simulink model "primer2"  (R2014a)
settings: Solver=ode45  StartTime=0.0  StopTime=50.0  RelTol=1e-3
undefined symbols (not defined in the file): des, gcbh
settings Model: Creator=Student  LastModifiedBy=almi0
settings OptimizationCC: ExpressionDepthLimit=2147483647
settings DebuggingCC: UnderspecifiedInitializationDetection=Classic  StateNameClashWarn=warning

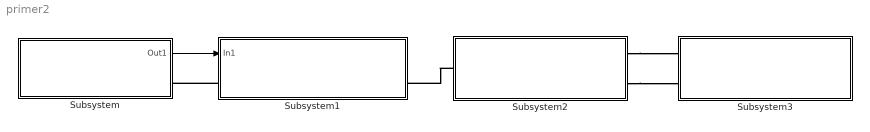
== system primer2 ==
  Subsystem : Subsystem
  Subsystem1 : Subsystem
  Subsystem2 : Subsystem
  Subsystem3 : Subsystem
  wires:
  Subsystem/1(Out1) -> Subsystem1/1(In1)
  connections:
  Subsystem1/LConn1 -- Subsystem/RConn1
  Subsystem2/LConn1 -- Subsystem1/RConn2
  Subsystem2/RConn1 -- Subsystem3/LConn1
  Subsystem2/RConn2 -- Subsystem3/LConn2

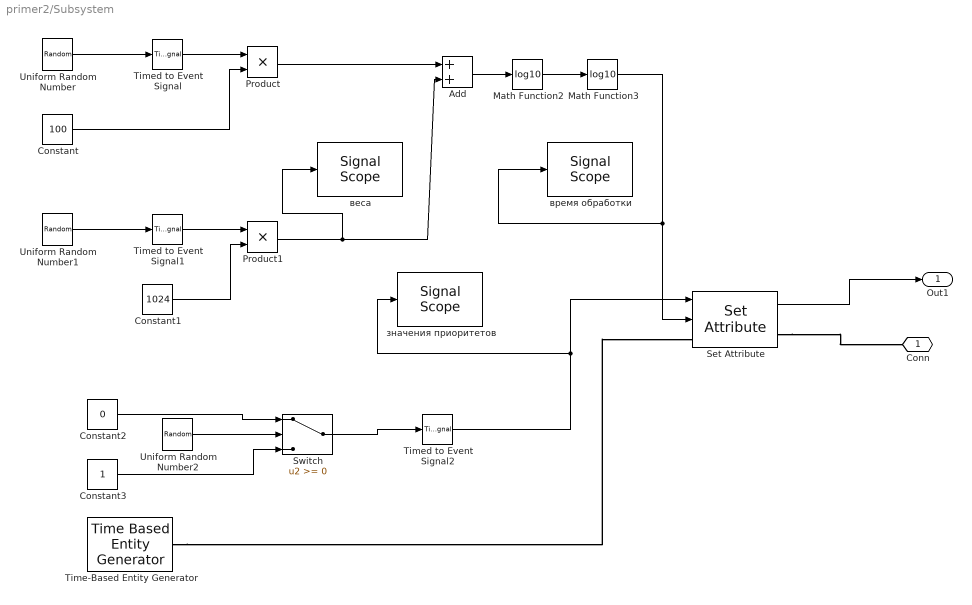
== system primer2/Subsystem ==
  Add : Sum
  Constant : Constant  Value=100
  Constant1 : Constant  Value=1024
  Constant2 : Constant  Value=0
  Constant3 : Constant
  Math Function2 : Math  Operator=log10  SaturateOnIntegerOverflow=on
  Math Function3 : Math  Operator=log10  SaturateOnIntegerOverflow=on
  Product : Product  RndMeth=Zero
  Product1 : Product  RndMeth=Zero
  Set Attribute : SetAttribute  AttributeName=Priority|ServTime  AttributeFrom=Signal port|Signal port  AttributeValue=1|1  AttributeTreatAsVector=1|1  StatNumberDeparted=on  EvaluatedAttributeValue={ [];[]}
      settings: InputPortMap=u0,u1
  Switch : Switch
  Time-Based Entity Generator : TimeBasedEntityGenerator
  Timed to Event Signal : TimedToEventSignal
  Timed to Event Signal1 : TimedToEventSignal
  Timed to Event Signal2 : TimedToEventSignal
  Uniform Random Number : UniformRandomNumber  Minimum=0  SampleTime=0.1
  Uniform Random Number1 : UniformRandomNumber  Minimum=0  SampleTime=0.1
  Uniform Random Number2 : UniformRandomNumber  Minimum=0  SampleTime=0.1
  веса : SignalScope  LoadFcn=des.scope.CallbackSupport('seLoadFcn',gcbh)  StartFcn=des.scope.CallbackSupport('seStartFcn',gcbh)  StopFcn=des.scope.CallbackSupport('seStopFcn',gcbh)
      settings: CopyFcn=des.scope.CallbackSupport('seCopyFcn',gcbh)  DeleteFcn=des.scope.CallbackSupport('seDeleteFcn',gcbh)  PreSaveFcn=des.scope.CallbackSupport('sePreSaveFcn',gcbh)  NameChangeFcn=des.scope.CallbackSupport('seNameChangeFcn',gcbh)  OpenFcn=des.scope.CallbackSupport('seOpenFcn',gcbh)
  время обработки : SignalScope  LoadFcn=des.scope.CallbackSupport('seLoadFcn',gcbh)  StartFcn=des.scope.CallbackSupport('seStartFcn',gcbh)  StopFcn=des.scope.CallbackSupport('seStopFcn',gcbh)  ShowCountPlotted=on
      settings: CopyFcn=des.scope.CallbackSupport('seCopyFcn',gcbh)  DeleteFcn=des.scope.CallbackSupport('seDeleteFcn',gcbh)  PreSaveFcn=des.scope.CallbackSupport('sePreSaveFcn',gcbh)  NameChangeFcn=des.scope.CallbackSupport('seNameChangeFcn',gcbh)  OpenFcn=des.scope.CallbackSupport('seOpenFcn',gcbh)
  значения приоритетов : SignalScope  LoadFcn=des.scope.CallbackSupport('seLoadFcn',gcbh)  StartFcn=des.scope.CallbackSupport('seStartFcn',gcbh)  StopFcn=des.scope.CallbackSupport('seStopFcn',gcbh)
      settings: CopyFcn=des.scope.CallbackSupport('seCopyFcn',gcbh)  DeleteFcn=des.scope.CallbackSupport('seDeleteFcn',gcbh)  PreSaveFcn=des.scope.CallbackSupport('sePreSaveFcn',gcbh)  NameChangeFcn=des.scope.CallbackSupport('seNameChangeFcn',gcbh)  OpenFcn=des.scope.CallbackSupport('seOpenFcn',gcbh)
  Conn : PMIOPort  Port=1  Side=Right
  Out1 : Outport
  wires:
  Switch/1 -> Timed to Event Signal2/1
  Constant2/1 -> Switch/1
  Set Attribute/1 -> Out1/1
  Constant/1 -> Product/2
  Uniform Random Number/1 -> Timed to Event Signal/1
  Math Function2/1 -> Math Function3/1
  Timed to Event Signal/1 -> Product/1
  Product1/1 -> веса/1, Add/2
  Product/1 -> Add/1
  Timed to Event Signal1/1 -> Product1/1
  Constant1/1 -> Product1/2
  Uniform Random Number1/1 -> Timed to Event Signal1/1
  Add/1 -> Math Function2/1
  Constant3/1 -> Switch/3
  Uniform Random Number2/1 -> Switch/2
  Timed to Event Signal2/1 -> Set Attribute/1, значения приоритетов/1
  Math Function3/1 -> время обработки/1, Set Attribute/2
  connections:
  Time-Based Entity Generator/RConn1 -- Set Attribute/LConn1
  Set Attribute/RConn1 -- Conn/RConn1

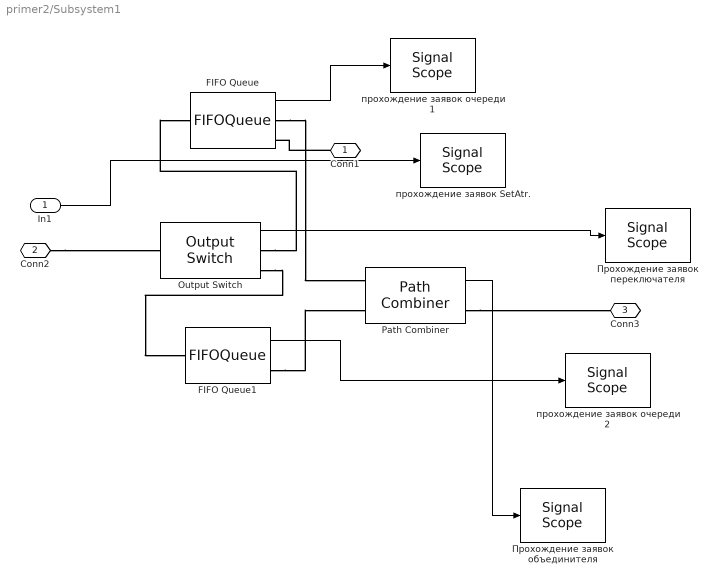
== system primer2/Subsystem1 ==
  In1 : Inport
  FIFO Queue : FIFOQueue  EnableTOPort=on  StatNumberDeparted=on
  FIFO Queue1 : FIFOQueue  StatNumberDeparted=on
  Output Switch : OutputSwitch  NumberOutputPorts=2  StatNumberDeparted=on
  Path Combiner : PathCombiner  NumberInputPorts=2  StatNumberDeparted=on
  Прохождение заявок объединителя : SignalScope  LoadFcn=des.scope.CallbackSupport('seLoadFcn',gcbh)  StartFcn=des.scope.CallbackSupport('seStartFcn',gcbh)  StopFcn=des.scope.CallbackSupport('seStopFcn',gcbh)
      settings: CopyFcn=des.scope.CallbackSupport('seCopyFcn',gcbh)  DeleteFcn=des.scope.CallbackSupport('seDeleteFcn',gcbh)  PreSaveFcn=des.scope.CallbackSupport('sePreSaveFcn',gcbh)  NameChangeFcn=des.scope.CallbackSupport('seNameChangeFcn',gcbh)  OpenFcn=des.scope.CallbackSupport('seOpenFcn',gcbh)
  Прохождение заявок переключателя : SignalScope  LoadFcn=des.scope.CallbackSupport('seLoadFcn',gcbh)  StartFcn=des.scope.CallbackSupport('seStartFcn',gcbh)  StopFcn=des.scope.CallbackSupport('seStopFcn',gcbh)
      settings: CopyFcn=des.scope.CallbackSupport('seCopyFcn',gcbh)  DeleteFcn=des.scope.CallbackSupport('seDeleteFcn',gcbh)  PreSaveFcn=des.scope.CallbackSupport('sePreSaveFcn',gcbh)  NameChangeFcn=des.scope.CallbackSupport('seNameChangeFcn',gcbh)  OpenFcn=des.scope.CallbackSupport('seOpenFcn',gcbh)
  прохождение заявок SetAtr. : SignalScope  LoadFcn=des.scope.CallbackSupport('seLoadFcn',gcbh)  StartFcn=des.scope.CallbackSupport('seStartFcn',gcbh)  StopFcn=des.scope.CallbackSupport('seStopFcn',gcbh)
      settings: CopyFcn=des.scope.CallbackSupport('seCopyFcn',gcbh)  DeleteFcn=des.scope.CallbackSupport('seDeleteFcn',gcbh)  PreSaveFcn=des.scope.CallbackSupport('sePreSaveFcn',gcbh)  NameChangeFcn=des.scope.CallbackSupport('seNameChangeFcn',gcbh)  OpenFcn=des.scope.CallbackSupport('seOpenFcn',gcbh)
  прохождение заявок очереди 1 : SignalScope  LoadFcn=des.scope.CallbackSupport('seLoadFcn',gcbh)  StartFcn=des.scope.CallbackSupport('seStartFcn',gcbh)  StopFcn=des.scope.CallbackSupport('seStopFcn',gcbh)
      settings: CopyFcn=des.scope.CallbackSupport('seCopyFcn',gcbh)  DeleteFcn=des.scope.CallbackSupport('seDeleteFcn',gcbh)  PreSaveFcn=des.scope.CallbackSupport('sePreSaveFcn',gcbh)  NameChangeFcn=des.scope.CallbackSupport('seNameChangeFcn',gcbh)  OpenFcn=des.scope.CallbackSupport('seOpenFcn',gcbh)
  прохождение заявок очереди 2 : SignalScope  LoadFcn=des.scope.CallbackSupport('seLoadFcn',gcbh)  StartFcn=des.scope.CallbackSupport('seStartFcn',gcbh)  StopFcn=des.scope.CallbackSupport('seStopFcn',gcbh)
      settings: CopyFcn=des.scope.CallbackSupport('seCopyFcn',gcbh)  DeleteFcn=des.scope.CallbackSupport('seDeleteFcn',gcbh)  PreSaveFcn=des.scope.CallbackSupport('sePreSaveFcn',gcbh)  NameChangeFcn=des.scope.CallbackSupport('seNameChangeFcn',gcbh)  OpenFcn=des.scope.CallbackSupport('seOpenFcn',gcbh)
  Conn1 : PMIOPort  Port=1  Side=Right
  Conn2 : PMIOPort  Port=2  Side=Left
  Conn3 : PMIOPort  Port=3  Side=Right
  wires:
  In1/1 -> прохождение заявок SetAtr./1
  FIFO Queue/1 -> прохождение заявок очереди 1/1
  FIFO Queue1/1 -> прохождение заявок очереди 2/1
  Output Switch/1 -> Прохождение заявок переключателя/1
  Path Combiner/1 -> Прохождение заявок объединителя/1
  connections:
  Path Combiner/RConn1 -- Conn3/RConn1
  Conn2/RConn1 -- Output Switch/LConn1
  Conn1/RConn1 -- FIFO Queue/RConn2
  Output Switch/RConn1 -- FIFO Queue/LConn1
  FIFO Queue/RConn1 -- Path Combiner/LConn1
  Output Switch/RConn2 -- FIFO Queue1/LConn1
  FIFO Queue1/RConn1 -- Path Combiner/LConn2

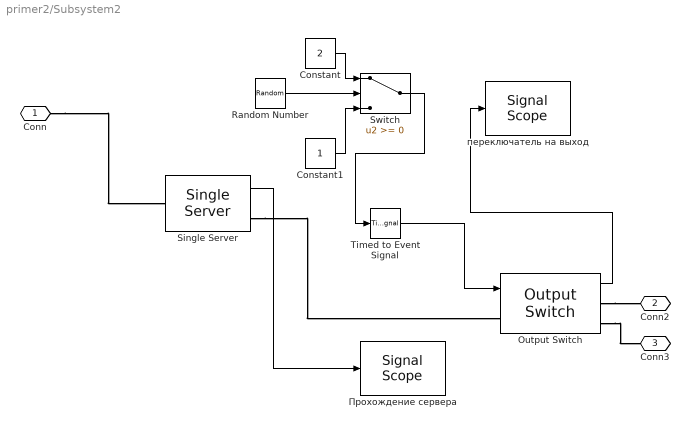
== system primer2/Subsystem2 ==
  Constant : Constant  Value=2
  Constant1 : Constant
  Output Switch : OutputSwitch  NumberOutputPorts=2  SwitchingCriterion=From signal port p  InitialConditions=2  StatNumberDeparted=on
  Random Number : RandomNumber  SampleTime=0.1
  Single Server : SingleServer  StatNumberDeparted=on
  Switch : Switch
  Timed to Event Signal : TimedToEventSignal
  Прохождение сервера : SignalScope  LoadFcn=des.scope.CallbackSupport('seLoadFcn',gcbh)  StartFcn=des.scope.CallbackSupport('seStartFcn',gcbh)  StopFcn=des.scope.CallbackSupport('seStopFcn',gcbh)
      settings: CopyFcn=des.scope.CallbackSupport('seCopyFcn',gcbh)  DeleteFcn=des.scope.CallbackSupport('seDeleteFcn',gcbh)  PreSaveFcn=des.scope.CallbackSupport('sePreSaveFcn',gcbh)  NameChangeFcn=des.scope.CallbackSupport('seNameChangeFcn',gcbh)  OpenFcn=des.scope.CallbackSupport('seOpenFcn',gcbh)
  переключатель на выход : SignalScope  LoadFcn=des.scope.CallbackSupport('seLoadFcn',gcbh)  StartFcn=des.scope.CallbackSupport('seStartFcn',gcbh)  StopFcn=des.scope.CallbackSupport('seStopFcn',gcbh)
      settings: CopyFcn=des.scope.CallbackSupport('seCopyFcn',gcbh)  DeleteFcn=des.scope.CallbackSupport('seDeleteFcn',gcbh)  PreSaveFcn=des.scope.CallbackSupport('sePreSaveFcn',gcbh)  NameChangeFcn=des.scope.CallbackSupport('seNameChangeFcn',gcbh)  OpenFcn=des.scope.CallbackSupport('seOpenFcn',gcbh)
  Conn : PMIOPort  Port=1  Side=Left
  Conn2 : PMIOPort  Port=2  Side=Right
  Conn3 : PMIOPort  Port=3  Side=Right
  wires:
  Single Server/1 -> Прохождение сервера/1
  Constant/1 -> Switch/1
  Output Switch/1 -> переключатель на выход/1
  Timed to Event Signal/1 -> Output Switch/1
  Random Number/1 -> Switch/2
  Constant1/1 -> Switch/3
  Switch/1 -> Timed to Event Signal/1
  connections:
  Conn/RConn1 -- Single Server/LConn1
  Single Server/RConn1 -- Output Switch/LConn1
  Output Switch/RConn1 -- Conn2/RConn1
  Output Switch/RConn2 -- Conn3/RConn1

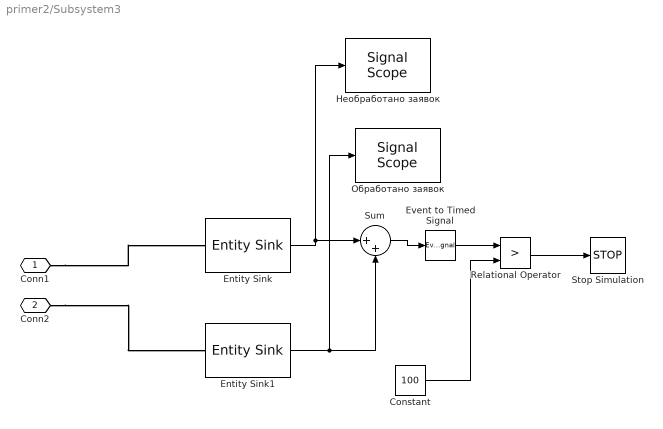
== system primer2/Subsystem3 ==
  Constant : Constant  Value=100
  Entity Sink : EntitySink  StatNumberArrived=on
  Entity Sink1 : EntitySink  StatNumberArrived=on
  Event to Timed Signal : EventToTimedSignal
  Relational Operator : RelationalOperator  Operator=>  OutDataTypeStr=boolean
  Stop Simulation : Stop
  Sum : Sum  Inputs=|++
  Необработано заявок : SignalScope  LoadFcn=des.scope.CallbackSupport('seLoadFcn',gcbh)  StartFcn=des.scope.CallbackSupport('seStartFcn',gcbh)  StopFcn=des.scope.CallbackSupport('seStopFcn',gcbh)
      settings: CopyFcn=des.scope.CallbackSupport('seCopyFcn',gcbh)  DeleteFcn=des.scope.CallbackSupport('seDeleteFcn',gcbh)  PreSaveFcn=des.scope.CallbackSupport('sePreSaveFcn',gcbh)  NameChangeFcn=des.scope.CallbackSupport('seNameChangeFcn',gcbh)  OpenFcn=des.scope.CallbackSupport('seOpenFcn',gcbh)
  Обработано заявок : SignalScope  LoadFcn=des.scope.CallbackSupport('seLoadFcn',gcbh)  StartFcn=des.scope.CallbackSupport('seStartFcn',gcbh)  StopFcn=des.scope.CallbackSupport('seStopFcn',gcbh)
      settings: CopyFcn=des.scope.CallbackSupport('seCopyFcn',gcbh)  DeleteFcn=des.scope.CallbackSupport('seDeleteFcn',gcbh)  PreSaveFcn=des.scope.CallbackSupport('sePreSaveFcn',gcbh)  NameChangeFcn=des.scope.CallbackSupport('seNameChangeFcn',gcbh)  OpenFcn=des.scope.CallbackSupport('seOpenFcn',gcbh)
  Conn1 : PMIOPort  Port=1  Side=Left
  Conn2 : PMIOPort  Port=2  Side=Left
  wires:
  Sum/1 -> Event to Timed Signal/1
  Entity Sink1/1 -> Обработано заявок/1, Sum/2
  Relational Operator/1 -> Stop Simulation/1
  Event to Timed Signal/1 -> Relational Operator/1
  Constant/1 -> Relational Operator/2
  Entity Sink/1 -> Необработано заявок/1, Sum/1
  connections:
  Conn1/RConn1 -- Entity Sink/LConn1
  Conn2/RConn1 -- Entity Sink1/LConn1
